simulink model "TSFS06lab1"  (R2018b)
settings: Solver=ode45  StartTime=0.0  StopTime=50.0  RelTol=1e-3  EnableMultiTasking=on
values from neighbouring files (symbols this model uses):
  alpha1 = 1    [labskel.m]
  alpha2 = 0.05    [labskel.m]
  alpha3 = 0.1    [labskel.m]
  alpha4 = 0.1    [labskel.m]
  f1 = 0    [labskel.m]
  f2 = 0    [labskel.m]
  f3 = 0    [labskel.m]
  f4 = 0    [labskel.m]
  Fc = ss(1/abs(evalfr(Fc*Gdes, 1i*wcdes))*Fc)    [controllerdesign.m]
  J1 = 1    [labskel.m]
  J2 = 0.5    [labskel.m]
  k = 99/90    (= 1.1)    [labskel.m]
  R = [R1;R2;R3;R4]    [labskel.m]    (also in tasks.m = Nh*L)
  Rseed = floor(sum(100*clock))    [labskel.m]
  Tfault = 25    [labskel.m]
libraries: simulink x3
settings Model: ExtModeTrigMode=oneshot  ExtModeArmWhenConnect=off  ExtModeAutoUpdateStatusClock=off  Creator=frisk  LastModifiedBy=Mattias Langsér
settings DataIOCC: SaveFormat=Array  SignalLoggingSaveFormat=ModelDataLogs
settings OptimizationCC: BlockReduction=off  BooleanDataType=off  ExpressionDepthLimit=2147483647  InitFltsAndDblsToZero=on  LifeSpan=inf
settings DebuggingCC: SaveWithParameterizedLinksMsg=none  UnderspecifiedInitializationDetection=Classic  MergeDetectMultiDrivingBlocksExec=none  SignalResolutionControl=TryResolveAllWithWarning  MultiTaskDSMMsg=warning  MultiTaskCondExecSysMsg=none  FcnCallInpInsideContextMsg=warning  StateNameClashWarn=warning  SFUnexpectedBacktrackingDiag=warning  SFNoUnconditionalDefaultTransitionDiag=warning  SFExecutionAtInitializationDiag=none
settings HardwareCC: ProdBitPerPointer=32  ProdBitPerSizeT=32  ProdBitPerPtrDiffT=32  ProdLargestAtomicFloat=None  ProdIntDivRoundTo=Undefined  ProdEndianess=Unspecified  ProdWordSize=32  ProdHWDeviceType=32-bit Generic  TargetUnknown=on
settings ModelReferenceCC: PropagateSignalLabelsOutOfModel=off
settings SFSimCC: SimUseLocalCustomCode=off
settings RTWCC: Description=Generic Real-Time Target  RTWUseLocalCustomCode=off
settings CodeAppCC: StateflowObjectComments=on
settings GRTTargetCC: TargetFcnLib=ansi_tfl_tmw.mat  TargetLangStandard=C89/C90 (ANSI)  GeneratePreprocessorConditionals=Disable all  CombineOutputUpdateFcns=off  GRTInterface=on
settings ConfigComp: CovMetricSettings=dw  CovHtmlReporting=on  CovSaveCumulativeToWorkspaceVar=on  CovSaveSingleToWorkspaceVar=on  CovExternalEMLEnable=off

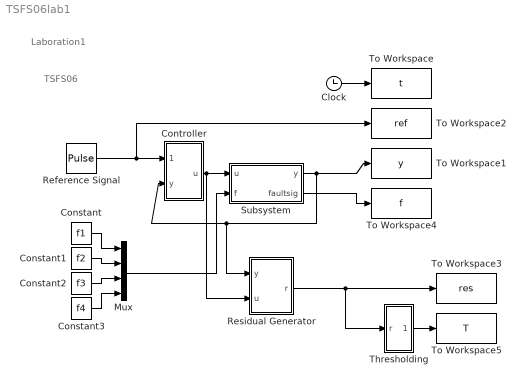
== system TSFS06lab1 ==
  note: Laboration1
  note: TSFS06
  Clock : Clock
  Constant : Constant  Value=f1
  Constant1 : Constant  Value=f2
  Constant2 : Constant  Value=f3
  Constant3 : Constant  Value=f4
  Controller : Subsystem
  Mux : Mux
  Reference Signal : DiscretePulseGenerator  Period=20  PulseWidth=10  PhaseDelay=1
  Residual Generator : Subsystem
  Subsystem : Subsystem
      mask Display:
      | disp('Flexible\n\n')
      | disp('Servo')
  Thresholding : Subsystem
  To Workspace : ToWorkspace  VariableName=t  SampleTime=0.1
  To Workspace1 : ToWorkspace  VariableName=y  SampleTime=0.1
  To Workspace2 : ToWorkspace  VariableName=ref  SampleTime=0.1
  To Workspace3 : ToWorkspace  VariableName=res  SampleTime=0.1
  To Workspace4 : ToWorkspace  VariableName=f  SampleTime=0.1
  To Workspace5 : ToWorkspace  VariableName=T  SampleTime=0.1
  wires:
  Reference Signal/1 -> Controller/1(ref), To Workspace2/1
  Subsystem/1(y) -> To Workspace1/1, Controller/2(y), Residual Generator/1(y)
  Controller/1(u) -> Subsystem/1(u), Residual Generator/2(u)
  Subsystem/2(faultsig) -> To Workspace4/1
  Thresholding/1(d) -> To Workspace5/1
  Mux/1 -> Subsystem/2(f)
  Constant2/1 -> Mux/3
  Constant1/1 -> Mux/2
  Constant/1 -> Mux/1
  Constant3/1 -> Mux/4
  Clock/1 -> To Workspace/1
  Residual Generator/1(r) -> To Workspace3/1, Thresholding/1(r)

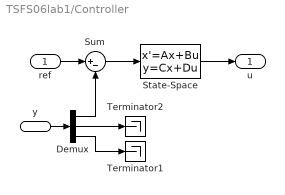
== system TSFS06lab1/Controller ==
  ref : Inport
  y : Inport  Port=2
  Demux : Demux  Outputs=3
  State-Space : StateSpace  A=Fc.a  B=Fc.b  C=Fc.c  D=Fc.d  InitialCondition=0
  Sum : Sum  Inputs=|+-  SaturateOnIntegerOverflow=on  InputSameDT=on  OutDataTypeStr=Inherit: Same as first input
  Terminator1 : Terminator
  Terminator2 : Terminator
  u : Outport
  wires:
  ref/1 -> Sum/1
  y/1 -> Demux/1
  Demux/1 -> Sum/2
  Demux/2 -> Terminator2/1
  Demux/3 -> Terminator1/1
  State-Space/1 -> u/1
  Sum/1 -> State-Space/1

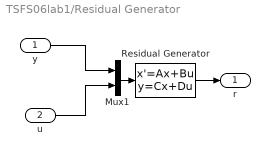
== system TSFS06lab1/Residual Generator ==
  y : Inport
  u : Inport  Port=2
  Mux1 : Mux  Inputs=2
  Residual Generator : StateSpace  A=R.a  B=R.b  C=R.c  D=R.d  InitialCondition=0
  r : Outport
  wires:
  u/1 -> Mux1/2
  y/1 -> Mux1/1
  Mux1/1 -> Residual Generator/1
  Residual Generator/1 -> r/1

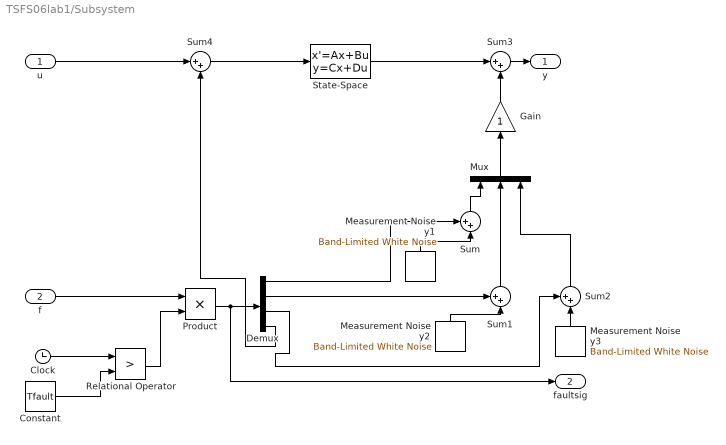
== system TSFS06lab1/Subsystem ==
  u : Inport
  f : Inport  Port=2
  Clock : Clock
  Constant : Constant  Value=Tfault
  Demux : Demux
  Gain : Gain  SaturateOnIntegerOverflow=on  OutDataTypeStr=Inherit: Same as input  ParamDataTypeStr=Inherit: Same as input
  Measurement Noise y1 : simulink/Sources/Band-Limited White Noise  Cov=NP  Ts=0.1  seed=Rseed
  Measurement Noise y2 : simulink/Sources/Band-Limited White Noise  Cov=NP  Ts=0.1  seed=Rseed+1
  Measurement Noise y3 : simulink/Sources/Band-Limited White Noise  Cov=NP  Ts=0.1  seed=Rseed+2
  Mux : Mux  Inputs=3
  Product : Product  SaturateOnIntegerOverflow=on  RndMeth=Zero  InputSameDT=on  OutDataTypeStr=Inherit: Same as first input
  Relational Operator : RelationalOperator  Operator=>  RndMeth=Nearest  InputSameDT=on
  State-Space : StateSpace  A=[0 1 0 0;-alpha2/J1 -(alpha1+alpha3)/J1 alpha2/J1 alpha3/J1;0 0 0 1;alpha2/J2 alpha3/J2 -alpha2/J2 -(alpha3+alpha4)/J2]  B=[0;k/J1;0;0]  C=[eye(3) zeros(3,1)]  D=zeros(3,1)  InitialCondition=zeros(4,1)
  Sum : Sum  Inputs=++|
  Sum1 : Sum  Inputs=++|
  Sum2 : Sum  Inputs=++|
  Sum3 : Sum  Inputs=|++  SaturateOnIntegerOverflow=on  InputSameDT=on  OutDataTypeStr=Inherit: Same as first input
  Sum4 : Sum  Inputs=|++
  y : Outport
  faultsig : Outport  Port=2
  wires:
  f/1 -> Product/1
  Relational Operator/1 -> Product/2
  Product/1 -> Demux/1, faultsig/1
  Sum3/1 -> y/1
  Clock/1 -> Relational Operator/1
  Constant/1 -> Relational Operator/2
  Gain/1 -> Sum3/2
  State-Space/1 -> Sum3/1
  Demux/1 -> Sum/1
  Demux/2 -> Sum1/1
  Demux/3 -> Sum2/1
  Demux/4 -> Sum4/2
  Mux/1 -> Gain/1
  Sum/1 -> Mux/1
  Measurement Noise y1/1 -> Sum/2
  Measurement Noise y3/1 -> Sum2/2
  Sum2/1 -> Mux/3
  Sum1/1 -> Mux/2
  Measurement Noise y2/1 -> Sum1/2
  Sum4/1 -> State-Space/1
  u/1 -> Sum4/1

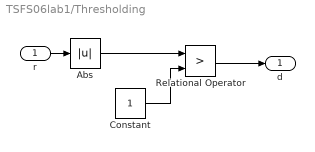
== system TSFS06lab1/Thresholding ==
  r : Inport
  Abs : Abs  SaturateOnIntegerOverflow=on
  Constant : Constant
  Relational Operator : RelationalOperator  Operator=>  RndMeth=Nearest  InputSameDT=on
  d : Outport
  wires:
  r/1 -> Abs/1
  Constant/1 -> Relational Operator/2
  Relational Operator/1 -> d/1
  Abs/1 -> Relational Operator/1
